simulink model "sensorCoreAlgorithm"  (R2022a)
settings: configuration reference "CommonConfigurationSet" (kept outside this file)
model workspace (MATLAB code in the model file + MAT data in the model file):
  cmdLim = Simulink.Parameter
  cmdLim.Value = 15
  cmdLim.Description = 'Limit for controlling the maximum surface command angle.'
  cmdLim.Min = 0
  cmdLim.Max = 90
  cmdLim.DocUnits = 'deg'
  dispGain = Simulink.Parameter
  dispGain.Value = 0.75
  dispGain.Description = 'Gain applied to the displacement error.'
  dispGain.Min = 0
  dispGain.Max = []
  dispGain.DocUnits = 'deg/sec/deg'
  dispLim = Simulink.Parameter
  dispLim.Value = 30
  dispLim.Description = 'Limit for controlling the maximum commanded angle.'
  dispLim.Min = 0
  dispLim.Max = 180
  dispLim.DocUnits = 'deg'
  intGain = Simulink.Parameter
  intGain.Value = 0.5
  intGain.Description = 'Gain applied to the integral error.'
  intGain.Min = 0
  intGain.Max = []
  intGain.DocUnits = 'deg/sec/deg/sec'
  intLim = Simulink.Parameter
  intLim.Value = 5
  intLim.Description = 'Limit for controlling the maximum commanded angle.'
  intLim.Min = 0
  intLim.Max = 90
  intLim.DocUnits = 'deg'
  rateGain = Simulink.Parameter
  rateGain.Value = 2
  rateGain.Description = 'Gain applied to the rate error.'
  rateGain.Min = 0
  rateGain.Max = []
  rateGain.DocUnits = 'deg/deg/sec'
  rateLim = Simulink.Parameter
  rateLim.Value = 6
  rateLim.Description = 'Limit for controlling the maximum commanded angle.'
  rateLim.Min = 0
  rateLim.Max = 180
  rateLim.DocUnits = 'deg/sec'
  hdgGain = Simulink.Parameter
  hdgGain.Value = 0.015
  LOCAL_DEVICE_ID = Simulink.Parameter
  LOCAL_DEVICE_ID.Value.device_id = [0; 0; 0; 0; 0; 0; 0; 0; 0; 0]
  LOCAL_DEVICE_ID.DataType = 'Bus: DeviceIDBusType'
  LOCAL_DEVICE_ID.Complexity = 'real'
  LOCAL_DEVICE_ID.Dimensions = [1 1]
settings Model: RequirementInfo={} %GIDa_fe9045fd_0412_4b6e_8206_617cc20e6fde  DataDictionary=sensorCoreAlgorithmData.sldd  EnableAccessToBaseWorkspace=off  FPTRunName=Active  ParameterArgumentNames=LOCAL_DEVICE_ID  Creator=The MathWorks, Inc.  LastModifiedBy=The MathWorks, Inc.
settings ConfigSetRef: SourceName=CommonConfigurationSet

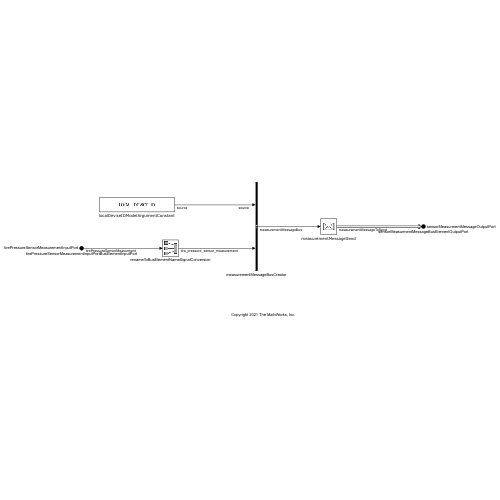
[thumbnail: Simulink's stored preview of the top-level diagram]
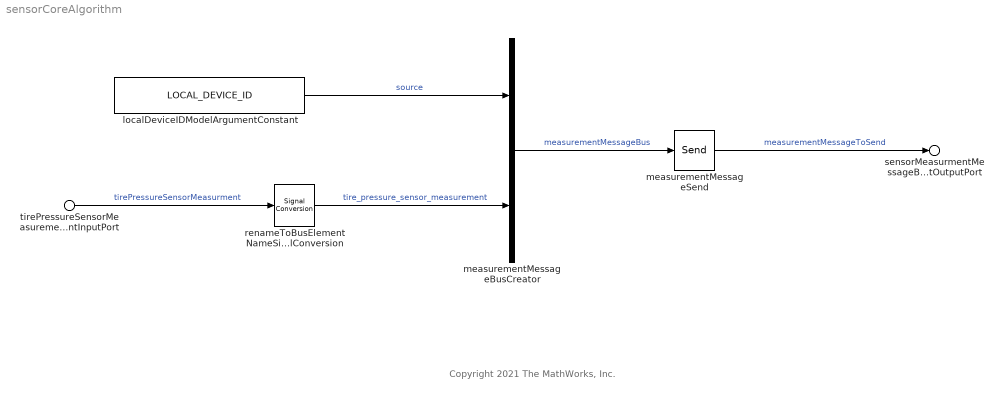
== system sensorCoreAlgorithm ==
  note: Copyright 2021 The MathWorks, Inc.
  tirePressureSensorMeasurementInputPortBusElementInputPort : Inport  PortName=tirePressureSensorMeasurementInputPort
  localDeviceIDModelArgumentConstant : Constant  Value=LOCAL_DEVICE_ID  OutDataTypeStr=Bus: DeviceIDBusType
  measurementMessageBusCreator : BusCreator  Inputs=2  OutDataTypeStr=Bus: MeasurementMsgBusType  NonVirtualBus=on
  measurementMessageSend : Send  OutputPortMessageModes=m
  renameToBusElementNameSignalConversion : SignalConversion  OverrideOpt=off
  sensorMeasurmentMessageBusElementOutputPort : Outport  InputPortMessageModes=m  PortName=sensorMeasurmentMessageOutputPort
  wires:
  tirePressureSensorMeasurementInputPortBusElementInputPort/1 -> renameToBusElementNameSignalConversion/1  "tirePressureSensorMeasurment"
  measurementMessageBusCreator/1 -> measurementMessageSend/1  "measurementMessageBus"
  localDeviceIDModelArgumentConstant/1 -> measurementMessageBusCreator/1  "source"
  measurementMessageSend/1 -> sensorMeasurmentMessageBusElementOutputPort/1  "measurementMessageToSend"
  renameToBusElementNameSignalConversion/1 -> measurementMessageBusCreator/2  "tire_pressure_sensor_measurement"
